simulink model "controller_dev_sg_HIL_noTP"  (R2018b)
settings: configuration reference "Physics" (kept outside this file)
model workspace (MAT data in the model file):
  m = 1000
values from neighbouring files (symbols this model uses):
  bool_activate_Vehicles : value not decoded    [controller_dev_sg.sldd]
  ModObj_ObjList_SendPort = 11004.0    [UDPPortConfig.sldd]
  ModSens_GpsSenDat_SendPort = 3002.0    [UDPPortConfig.sldd]
  sensors_freq_camera = 37.0    [controller_dev_sg.sldd]
  sensors_freq_gps = 20.0    [controller_dev_sg.sldd]
  sensors_freq_imu = 100.0    [controller_dev_sg.sldd]
  sensors_freq_lidar = 12.0    [controller_dev_sg.sldd]
  sensors_freq_radar = 20.0    [controller_dev_sg.sldd]
undefined symbols (not defined in the file or in its folder): activate_VariableFriction, C, tpa_map_Reference, tSPhysics, x0_vehiclepos_start_veh1, x0_vehiclepos_start_veh10, x0_vehiclepos_start_veh2, x0_vehiclepos_start_veh3, x0_vehiclepos_start_veh4, x0_vehiclepos_start_veh5, x0_vehiclepos_start_veh6, x0_vehiclepos_start_veh7, x0_vehiclepos_start_veh8, x0_vehiclepos_start_veh9
libraries: xpcutilitieslib x273, xpcrtudplib x215, aerolibconvert2 x48, simulink x30, etargetslib x26, speedgoatlib_IO612 x7, canmsglib x6, slrtlib x4
(part 1 of 16)
settings Model: DataDictionary=controller_dev_sg.sldd  sg_rtwmakecfg_data=_sglibc__IO61X_Library_  PauseTimes=9.280  Creator=wischnewski  LastModifiedBy=ga96wud

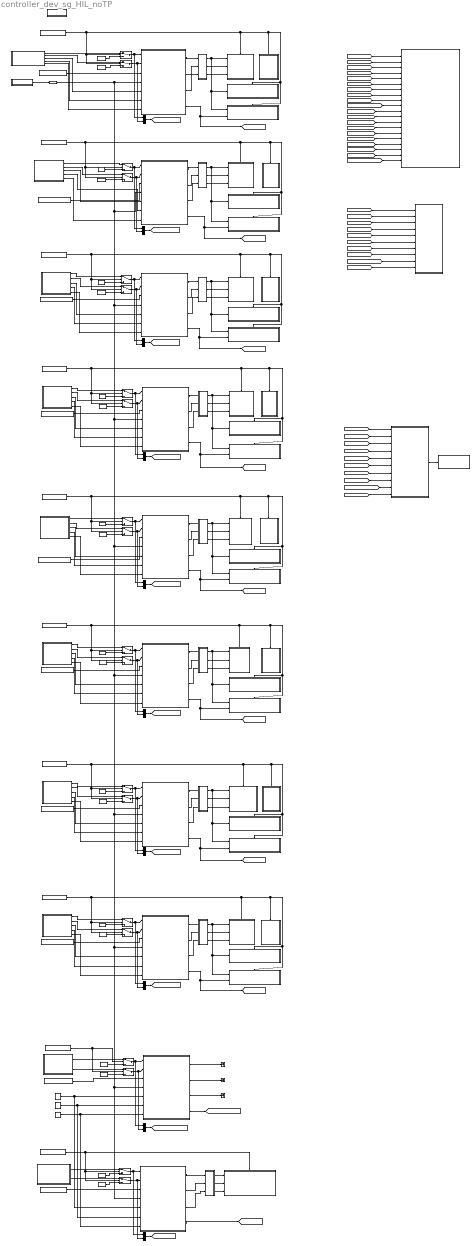
== system controller_dev_sg_HIL_noTP ==
  note: UDP to Object Detection (Object List)
  note: Roborace Vehicle on Nvidia and Speedgoat Mobile
  note: Author: Alexander Wischnewski (alexander.wischnewski@tum.de)
      | Chair of Automatic Control at TU Munich
      |
      | Description: This model uses the control software provided in vehicle dynamics control and the nonlinear single track vehicle model
      | with sensor models to simulate the example vehicle in closed loop.
  note: UDP to Unity Environment Simulation (Vehicle States)
  note: Dallara 1
  note: Configuration of Speedgoat Scopes
  note: Dallara 2
  note: Manual Steering
  note: Dallara 3
  note: Dallara 4
  note: Dallara 5
  note: Dallara 6
  note: Dallara 7
  note: Dallara 8
  Constant{,2,6,8..9,13,17,21..22,25,28,31..32} (13 alike) : Constant  Value=0
  Constant{1,3,10,12,14,18..19,23,26,29} (10 alike) : Constant  Value=-1000
  Constant11 : Constant  Value=bool_activate_Vehicles(1)  OutDataTypeStr=boolean
  Constant15 : Constant  Value=bool_activate_Vehicles(10)  OutDataTypeStr=boolean
  Constant16 : Constant  Value=bool_activate_Vehicles(3)  OutDataTypeStr=boolean
  Constant20 : Constant  Value=bool_activate_Vehicles(4)  OutDataTypeStr=boolean
  Constant24 : Constant  Value=bool_activate_Vehicles(6)  OutDataTypeStr=boolean
  Constant27 : Constant  Value=bool_activate_Vehicles(7)  OutDataTypeStr=boolean
  Constant30 : Constant  Value=bool_activate_Vehicles(8)  OutDataTypeStr=boolean
  Constant4 : Constant  Value=bool_activate_Vehicles(2)  OutDataTypeStr=boolean
  Constant5 : Constant  Value=bool_activate_Vehicles(9)  OutDataTypeStr=boolean
  Constant7 : Constant  Value=bool_activate_Vehicles(5)  OutDataTypeStr=boolean
  EnvironmentSim_Communication : Subsystem
  HardwareSetup : Subsystem
  Model{,1..8} (9 alike) : ModelReference  ModelNameDialog=convert_SimBus.slx  SimulationMode=Normal  ModelReferenceVersion=1.823
  Mux{,1..9} (10 alike) : Mux  Inputs=2
  Object List Preparation : Subsystem
  PassengerVehicle -  Manual Steering : ModelReference  ModelNameDialog=PassengerVehicle  SimulationMode=Normal  ModelReferenceVersion=1.994
  PassengerVehicle - Dallara {1..8} (8 alike) : ModelReference  ModelNameDialog=PassengerVehicle  SimulationMode=Normal  ModelReferenceVersion=1.994
  PassengerVehicle - Roborace : ModelReference  ModelNameDialog=PassengerVehicle  SimulationMode=Normal  ModelReferenceVersion=1.994
  Raptor State Machine 1 : Subsystem
  Raptor State Machine 2 : Subsystem
  Raptor State Machine 3 : Subsystem
  Raptor State Machine 4 : Subsystem
  Raptor State Machine 5 : Subsystem
  Raptor State Machine 6 : Subsystem
  Raptor State Machine 7 : Subsystem
  Raptor State Machine 8 : Subsystem
  Rate Transition5 : RateTransition
  Rx_VehicleControlCAN : Subsystem
  SpeedgoatScopes : Subsystem
  Subsystem1 : Subsystem
  Subsystem4 : Subsystem
  Switch{1..20} (20 alike) : Switch  Criteria=u2 > Threshold  Threshold=0.5
  Terminator3 : Terminator
  Terminator4 : Terminator
  Terminator5 : Terminator
  Tx_VehicleDataCAN : Subsystem
  "UDP from Control (Request for Steering Angle, Long. Force)" : Subsystem
  "UDP from Control (Request for Steering Angle, Long. Force)1" : Subsystem
  "UDP from Control (Request for Steering Angle, Long. Force)2" : Subsystem
  "UDP from Control (Request for Steering Angle, Long. Force)3" : Subsystem
  "UDP from Control (Request for Steering Angle, Long. Force)4" : Subsystem
  "UDP from Control (Request for Steering Angle, Long. Force)5" : Subsystem
  "UDP from Control (Request for Steering Angle, Long. Force)6" : Subsystem
  "UDP from Control (Request for Steering Angle, Long. Force)7" : Subsystem
  "UDP to Control (Position, IMU, Wheelspeed)" : Subsystem
  "UDP to Control (Position, IMU, Wheelspeed)1" : Subsystem
  "UDP to Control (Position, IMU, Wheelspeed)2" : Subsystem
  "UDP to Control (Position, IMU, Wheelspeed)3" : Subsystem
  "UDP to Control (Position, IMU, Wheelspeed)4" : Subsystem
  "UDP to Control (Position, IMU, Wheelspeed)5" : Subsystem
  "UDP to Control (Position, IMU, Wheelspeed)6" : Subsystem
  "UDP to Control (Position, IMU, Wheelspeed)7" : Subsystem
  "UDP to Mapping and Localization (Position, IMU, Wheelspeed)" : Subsystem
  "UDP to Mapping and Localization (Position, IMU, Wheelspeed)1" : Subsystem
  "UDP to Mapping and Localization (Position, IMU, Wheelspeed)2" : Subsystem
  "UDP to Mapping and Localization (Position, IMU, Wheelspeed)3" : Subsystem
  "UDP to Mapping and Localization (Position, IMU, Wheelspeed)4" : Subsystem
  "UDP to Mapping and Localization (Position, IMU, Wheelspeed)5" : Subsystem
  "UDP to Mapping and Localization (Position, IMU, Wheelspeed)6" : Subsystem
  "UDP to Mapping and Localization (Position, IMU, Wheelspeed)7" : Subsystem
  UDP to Object Detection : Subsystem
  "UDP to Sensors (GNSS, IMU)" : Subsystem
  "UDP to Sensors (GNSS, IMU)1" : Subsystem
  "UDP to Sensors (GNSS, IMU)2" : Subsystem
  "UDP to Sensors (GNSS, IMU)3" : Subsystem
  "UDP to Sensors (GNSS, IMU)4" : Subsystem
  "UDP to Sensors (GNSS, IMU)5" : Subsystem
  "UDP to Sensors (GNSS, IMU)6" : Subsystem
  "UDP to Sensors (GNSS, IMU)7" : Subsystem
  x0_Dallara1 : Constant  Value=[x0_vehiclepos_start_veh1 1]  VectorParams1D=off
  x0_Dallara2 : Constant  Value=[x0_vehiclepos_start_veh2 1]
  x0_Dallara3 : Constant  Value=[x0_vehiclepos_start_veh3 1]
  x0_Dallara4 : Constant  Value=[x0_vehiclepos_start_veh4 1]
  x0_Dallara5 : Constant  Value=[x0_vehiclepos_start_veh5 1]
  x0_Dallara6 : Constant  Value=[x0_vehiclepos_start_veh6 1]
  x0_Dallara7 : Constant  Value=[x0_vehiclepos_start_veh7 1]
  x0_Dallara8 : Constant  Value=[x0_vehiclepos_start_veh8 1]
  x0_DevBot : Constant  Value=[x0_vehiclepos_start_veh10 1]
  x0_ManSteer : Constant  Value=[x0_vehiclepos_start_veh9 1]
  wires:
  PassengerVehicle - Roborace/1 -> Model/1
  PassengerVehicle - Roborace/2 -> Model/2
  PassengerVehicle - Roborace/3 -> Model/3
  PassengerVehicle - Roborace/4 -> [SimRealState_RR]
  Switch3/1 -> Mux/1, PassengerVehicle - Roborace/1
  Switch5/1 -> Mux/2, PassengerVehicle - Roborace/2
  Rx_VehicleControlCAN/2(TractionForceSummedAtWheels_N) -> Switch5/1
  Constant15/1 -> Switch5/2, Switch3/2, Tx_VehicleDataCAN/Enable
  Model1/1 -> "UDP to Sensors (GNSS, IMU)"/1(VehicleSensorData), "UDP to Mapping and Localization (Position, IMU, Wheelspeed)"/1(VehicleSensorData), "UDP to Control (Position, IMU, Wheelspeed)"/1(VehicleSensorData)
  x0_Dallara2/1 -> PassengerVehicle - Dallara 2/3
  x0_ManSteer/1 -> PassengerVehicle -  Manual Steering/3
  x0_Dallara1/1 -> PassengerVehicle - Dallara 1/3
  Constant17/1 -> Switch3/3
  x0_DevBot/1 -> PassengerVehicle - Roborace/3
  Constant18/1 -> Switch5/3
  PassengerVehicle - Dallara 1/4 -> "UDP to Sensors (GNSS, IMU)"/2(SimRealState), [SimRealState_Dallara1]
  PassengerVehicle - Dallara 2/4 -> "UDP to Sensors (GNSS, IMU)1"/2(SimRealState), [SimRealState_Dallara2]
  PassengerVehicle -  Manual Steering/4 -> [SimRealState_ManualSteering]
  [SimRealState_RR] -> Object List Preparation/10(SimRealState_RR)
  [SimRealState_Dallara1] -> Object List Preparation/1(SimRealState_Dallara1)
  [SimRealState_Dallara2] -> Object List Preparation/2(SimRealState_Dallara2)
  [SimRealState_Dallara3] -> Object List Preparation/3(SimRealState_Dallara3)
  Model2/3 -> "UDP to Control (Position, IMU, Wheelspeed)1"/3(ActuatorLimitations)
  Model2/1 -> "UDP to Sensors (GNSS, IMU)1"/1(VehicleSensorData), "UDP to Mapping and Localization (Position, IMU, Wheelspeed)1"/1(VehicleSensorData), "UDP to Control (Position, IMU, Wheelspeed)1"/1(VehicleSensorData)
  Model2/2 -> "UDP to Control (Position, IMU, Wheelspeed)1"/2(VehicleSystemStatus)
  PassengerVehicle -  Manual Steering/3 -> Terminator3/1
  PassengerVehicle -  Manual Steering/2 -> Terminator5/1
  PassengerVehicle -  Manual Steering/1 -> Terminator4/1
  Object List Preparation/1(Objects) -> UDP to Object Detection/1(Objects)
  [SimRealState_RR] -> EnvironmentSim_Communication/10(SimRealState_RR)
  [SimRealState_Dallara1] -> EnvironmentSim_Communication/1(SimRealState_Dallara1)
  [SimRealState_Dallara2] -> EnvironmentSim_Communication/2(SimRealState_Dallara2)
  [SimRealState_Dallara3] -> EnvironmentSim_Communication/3(SimRealState_Dallara3)
  Constant3/1 -> Switch4/3
  Constant2/1 -> Switch2/3
  "UDP from Control (Request for Steering Angle, Long. Force)1"/1(SteeringAngleAtWheel_rad) -> Switch2/1
  "UDP from Control (Request for Steering Angle, Long. Force)1"/2(TractionForceSummedAtWheels_N) -> Switch4/1
  [SimRealState_RR] -> SpeedgoatScopes/1(SimRealState_RoboraceDB)
  [SimRealState_Dallara3] -> SpeedgoatScopes/4(SimRealState_Dallara3)
  [SimRealState_Dallara2] -> SpeedgoatScopes/3(SimRealState_Dallara2)
  [SimRealState_Dallara1] -> SpeedgoatScopes/2(SimRealState_Dallara1)
  Mux/1 -> [ControlCommand_RR]
  Mux1/1 -> [ControlCommand_Dallara1]
  Switch7/1 -> Mux1/1, PassengerVehicle - Dallara 1/1
  Switch1/1 -> Mux1/2, PassengerVehicle - Dallara 1/2
  Mux2/1 -> [ControlCommand_Dallara2]
  Switch4/1 -> Mux2/2, PassengerVehicle - Dallara 2/2
  Switch2/1 -> Mux2/1, PassengerVehicle - Dallara 2/1
  Mux3/1 -> [ControlCommand_ManualSteering]
  [ControlCommand_RR] -> SpeedgoatScopes/11(ControlCommand_RoboraceDB)
  [ControlCommand_Dallara1] -> SpeedgoatScopes/12(ControlCommand_Dallara1)
  [ControlCommand_Dallara2] -> SpeedgoatScopes/13(ControlCommand_Dallara2)
  [ControlCommand_Dallara3] -> SpeedgoatScopes/14(ControlCommand_Dallara3)
  Subsystem1/1(in_tpamapReference) -> Rate Transition5/1
  Rate Transition5/1 -> PassengerVehicle - Dallara 2/4, PassengerVehicle - Dallara 3/4, PassengerVehicle - Dallara 4/4, PassengerVehicle - Dallara 5/4, PassengerVehicle - Dallara 6/4, PassengerVehicle - Dallara 7/4, PassengerVehicle - Roborace/4, PassengerVehicle -  Manual Steering/4, PassengerVehicle - Dallara 8/4, PassengerVehicle - Dallara 1/4
  Constant11/1 -> Switch1/2, Switch7/2, "UDP to Sensors (GNSS, IMU)"/Enable, "UDP to Mapping and Localization (Position, IMU, Wheelspeed)"/Enable, Raptor State Machine 1/Enable, "UDP to Control (Position, IMU, Wheelspeed)"/Enable
  Model/1 -> Tx_VehicleDataCAN/1(VehicleSensorData)
  Model/3 -> Tx_VehicleDataCAN/3(ActuatorLimitations)
  Model/2 -> Tx_VehicleDataCAN/2(VehicleSystemStatus)
  PassengerVehicle - Dallara 1/2 -> Model1/2
  PassengerVehicle - Dallara 1/3 -> Model1/3
  Model1/3 -> "UDP to Control (Position, IMU, Wheelspeed)"/3(ActuatorLimitations)
  Model1/2 -> "UDP to Control (Position, IMU, Wheelspeed)"/2(VehicleSystemStatus)
  PassengerVehicle - Dallara 1/1 -> Model1/1
  PassengerVehicle - Dallara 2/3 -> Model2/3
  PassengerVehicle - Dallara 2/2 -> Model2/2
  PassengerVehicle - Dallara 2/1 -> Model2/1
  Rx_VehicleControlCAN/1(SteeringAngleAtWheel_rad) -> Switch3/1
  Switch12/1 -> Mux3/1, PassengerVehicle -  Manual Steering/1
  Switch13/1 -> Mux3/2, PassengerVehicle -  Manual Steering/2
  Constant6/1 -> Switch7/3
  Constant14/1 -> Switch1/3
  "UDP from Control (Request for Steering Angle, Long. Force)"/1(SteeringAngleAtWheel_rad) -> Switch7/1
  "UDP from Control (Request for Steering Angle, Long. Force)"/2(TractionForceSummedAtWheels_N) -> Switch1/1
  Constant/1 -> PassengerVehicle -  Manual Steering/5, PassengerVehicle - Roborace/5
  Constant8/1 -> PassengerVehicle -  Manual Steering/6, PassengerVehicle - Roborace/6
  Mux4/1 -> [ControlCommand_Dallara3]
  Model3/3 -> "UDP to Control (Position, IMU, Wheelspeed)2"/3(ActuatorLimitations)
  Model3/2 -> "UDP to Control (Position, IMU, Wheelspeed)2"/2(VehicleSystemStatus)
  PassengerVehicle - Dallara 3/1 -> Model3/1
  Constant16/1 -> Raptor State Machine 3/Enable, "UDP to Sensors (GNSS, IMU)2"/Enable, "UDP to Mapping and Localization (Position, IMU, Wheelspeed)2"/Enable, "UDP to Control (Position, IMU, Wheelspeed)2"/Enable, Switch9/2, Switch8/2
  PassengerVehicle - Dallara 3/2 -> Model3/2
  Switch8/1 -> Mux4/1, PassengerVehicle - Dallara 3/1
  PassengerVehicle - Dallara 3/3 -> Model3/3
  Switch9/1 -> Mux4/2, PassengerVehicle - Dallara 3/2
  Constant9/1 -> Switch8/3
  "UDP from Control (Request for Steering Angle, Long. Force)2"/2(TractionForceSummedAtWheels_N) -> Switch9/1
  Constant12/1 -> Switch9/3
  PassengerVehicle - Dallara 3/4 -> "UDP to Sensors (GNSS, IMU)2"/2(SimRealState), [SimRealState_Dallara3]
  x0_Dallara3/1 -> PassengerVehicle - Dallara 3/3
  Constant21/1 -> Switch10/3
  x0_Dallara4/1 -> PassengerVehicle - Dallara 4/3
  Switch11/1 -> Mux5/2, PassengerVehicle - Dallara 4/2
  PassengerVehicle - Dallara 4/4 -> "UDP to Sensors (GNSS, IMU)3"/2(SimRealState), [SimRealState_Dallara4]
  "UDP from Control (Request for Steering Angle, Long. Force)4"/2(TractionForceSummedAtWheels_N) -> Switch11/1
  Switch10/1 -> Mux5/1, PassengerVehicle - Dallara 4/1
  Model4/1 -> "UDP to Sensors (GNSS, IMU)3"/1(VehicleSensorData), "UDP to Mapping and Localization (Position, IMU, Wheelspeed)3"/1(VehicleSensorData), "UDP to Control (Position, IMU, Wheelspeed)3"/1(VehicleSensorData)
  PassengerVehicle - Dallara 4/2 -> Model4/2
  PassengerVehicle - Dallara 4/3 -> Model4/3
  Mux5/1 -> [ControlCommand_Dallara4]
  "UDP from Control (Request for Steering Angle, Long. Force)4"/1(SteeringAngleAtWheel_rad) -> Switch10/1
  Model4/2 -> "UDP to Control (Position, IMU, Wheelspeed)3"/2(VehicleSystemStatus)
  Model4/3 -> "UDP to Control (Position, IMU, Wheelspeed)3"/3(ActuatorLimitations)
  Constant19/1 -> Switch11/3
  PassengerVehicle - Dallara 4/1 -> Model4/1
  [SimRealState_Dallara4] -> SpeedgoatScopes/5(SimRealState_Dallara4)
  [ControlCommand_Dallara4] -> SpeedgoatScopes/15(ControlCommand_Dallara4)
  [SimRealState_Dallara4] -> EnvironmentSim_Communication/4(SimRealState_Dallara4)
  [SimRealState_Dallara4] -> Object List Preparation/4(SimRealState_Dallara4)
  Constant10/1 -> Switch13/3
  Constant5/1 -> Switch12/2, Switch13/2
  Subsystem4/1(SteeringWheelAngle_rad) -> Switch12/1
  Constant13/1 -> Switch12/3
  Subsystem4/2(TractionForceSummedAtWheels_N) -> Switch13/1
  "UDP from Control (Request for Steering Angle, Long. Force)"/3(ThrottleRequest_perc) -> PassengerVehicle - Dallara 1/5
  "UDP from Control (Request for Steering Angle, Long. Force)"/4(GearRequest) -> PassengerVehicle - Dallara 1/6
  "UDP from Control (Request for Steering Angle, Long. Force)"/5(BrakeRequest_bar) -> PassengerVehicle - Dallara 1/7
  "UDP from Control (Request for Steering Angle, Long. Force)1"/3(ThrottleRequest_perc) -> PassengerVehicle - Dallara 2/5
  "UDP from Control (Request for Steering Angle, Long. Force)1"/4(GearRequest) -> PassengerVehicle - Dallara 2/6
  "UDP from Control (Request for Steering Angle, Long. Force)1"/5(BrakeRequest_bar) -> PassengerVehicle - Dallara 2/7
  "UDP from Control (Request for Steering Angle, Long. Force)2"/1(SteeringAngleAtWheel_rad) -> Switch8/1
  "UDP from Control (Request for Steering Angle, Long. Force)2"/3(ThrottleRequest_perc) -> PassengerVehicle - Dallara 3/5
  "UDP from Control (Request for Steering Angle, Long. Force)2"/4(GearRequest) -> PassengerVehicle - Dallara 3/6
  "UDP from Control (Request for Steering Angle, Long. Force)2"/5(BrakeRequest_bar) -> PassengerVehicle - Dallara 3/7
  "UDP from Control (Request for Steering Angle, Long. Force)4"/3(ThrottleRequest_perc) -> PassengerVehicle - Dallara 4/5
  "UDP from Control (Request for Steering Angle, Long. Force)4"/4(GearRequest) -> PassengerVehicle - Dallara 4/6
  "UDP from Control (Request for Steering Angle, Long. Force)4"/5(BrakeRequest_bar) -> PassengerVehicle - Dallara 4/7
  PassengerVehicle - Dallara 5/4 -> "UDP to Sensors (GNSS, IMU)4"/2(SimRealState), [SimRealState_Dallara5]
  PassengerVehicle - Dallara 5/2 -> Model5/2
  "UDP from Control (Request for Steering Angle, Long. Force)3"/3(ThrottleRequest_perc) -> PassengerVehicle - Dallara 5/5
  Constant22/1 -> Switch6/3
  "UDP from Control (Request for Steering Angle, Long. Force)3"/5(BrakeRequest_bar) -> PassengerVehicle - Dallara 5/7
  Model5/2 -> "UDP to Control (Position, IMU, Wheelspeed)4"/2(VehicleSystemStatus)
  Constant7/1 -> Raptor State Machine 5/Enable, "UDP to Sensors (GNSS, IMU)4"/Enable, "UDP to Mapping and Localization (Position, IMU, Wheelspeed)4"/Enable, "UDP to Control (Position, IMU, Wheelspeed)4"/Enable, Switch14/2, Switch6/2
  Model5/3 -> "UDP to Control (Position, IMU, Wheelspeed)4"/3(ActuatorLimitations)
  PassengerVehicle - Dallara 5/3 -> Model5/3
  Mux6/1 -> [ControlCommand_Dallara5]
  Switch6/1 -> Mux6/1, PassengerVehicle - Dallara 5/1
  Model5/1 -> "UDP to Control (Position, IMU, Wheelspeed)4"/1(VehicleSensorData), "UDP to Sensors (GNSS, IMU)4"/1(VehicleSensorData), "UDP to Mapping and Localization (Position, IMU, Wheelspeed)4"/1(VehicleSensorData)
  Constant1/1 -> Switch14/3
  "UDP from Control (Request for Steering Angle, Long. Force)3"/1(SteeringAngleAtWheel_rad) -> Switch6/1
  "UDP from Control (Request for Steering Angle, Long. Force)3"/4(GearRequest) -> PassengerVehicle - Dallara 5/6
  PassengerVehicle - Dallara 5/1 -> Model5/1
  Switch14/1 -> Mux6/2, PassengerVehicle - Dallara 5/2
  x0_Dallara5/1 -> PassengerVehicle - Dallara 5/3
  "UDP from Control (Request for Steering Angle, Long. Force)3"/2(TractionForceSummedAtWheels_N) -> Switch14/1
  PassengerVehicle - Dallara 6/4 -> "UDP to Sensors (GNSS, IMU)5"/2(SimRealState), [SimRealState_Dallara6]
  PassengerVehicle - Dallara 6/2 -> Model6/2
  "UDP from Control (Request for Steering Angle, Long. Force)5"/3(ThrottleRequest_perc) -> PassengerVehicle - Dallara 6/5
  Constant25/1 -> Switch15/3
  "UDP from Control (Request for Steering Angle, Long. Force)5"/5(BrakeRequest_bar) -> PassengerVehicle - Dallara 6/7
  Model6/2 -> "UDP to Control (Position, IMU, Wheelspeed)5"/2(VehicleSystemStatus)
  Constant24/1 -> Raptor State Machine 6/Enable, "UDP to Sensors (GNSS, IMU)5"/Enable, "UDP to Mapping and Localization (Position, IMU, Wheelspeed)5"/Enable, "UDP to Control (Position, IMU, Wheelspeed)5"/Enable, Switch16/2, Switch15/2
  Model6/3 -> "UDP to Control (Position, IMU, Wheelspeed)5"/3(ActuatorLimitations)
  PassengerVehicle - Dallara 6/3 -> Model6/3
  Mux7/1 -> [ControlCommand_Dallara6]
  Switch15/1 -> Mux7/1, PassengerVehicle - Dallara 6/1
  Model6/1 -> "UDP to Control (Position, IMU, Wheelspeed)5"/1(VehicleSensorData), "UDP to Sensors (GNSS, IMU)5"/1(VehicleSensorData), "UDP to Mapping and Localization (Position, IMU, Wheelspeed)5"/1(VehicleSensorData)
  Constant23/1 -> Switch16/3
  "UDP from Control (Request for Steering Angle, Long. Force)5"/1(SteeringAngleAtWheel_rad) -> Switch15/1
  "UDP from Control (Request for Steering Angle, Long. Force)5"/4(GearRequest) -> PassengerVehicle - Dallara 6/6
  PassengerVehicle - Dallara 6/1 -> Model6/1
  Switch16/1 -> Mux7/2, PassengerVehicle - Dallara 6/2
  x0_Dallara6/1 -> PassengerVehicle - Dallara 6/3
  "UDP from Control (Request for Steering Angle, Long. Force)5"/2(TractionForceSummedAtWheels_N) -> Switch16/1
  PassengerVehicle - Dallara 7/4 -> "UDP to Sensors (GNSS, IMU)6"/2(SimRealState), [SimRealState_Dallara7]
  PassengerVehicle - Dallara 7/2 -> Model7/2
  "UDP from Control (Request for Steering Angle, Long. Force)6"/3(ThrottleRequest_perc) -> PassengerVehicle - Dallara 7/5
  Constant28/1 -> Switch17/3
  "UDP from Control (Request for Steering Angle, Long. Force)6"/5(BrakeRequest_bar) -> PassengerVehicle - Dallara 7/7
  Model7/2 -> "UDP to Control (Position, IMU, Wheelspeed)6"/2(VehicleSystemStatus)
  Constant27/1 -> Raptor State Machine 7/Enable, "UDP to Sensors (GNSS, IMU)6"/Enable, "UDP to Mapping and Localization (Position, IMU, Wheelspeed)6"/Enable, "UDP to Control (Position, IMU, Wheelspeed)6"/Enable, Switch18/2, Switch17/2
  Model7/3 -> "UDP to Control (Position, IMU, Wheelspeed)6"/3(ActuatorLimitations)
  PassengerVehicle - Dallara 7/3 -> Model7/3
  Mux8/1 -> [ControlCommand_Dallara7]
  Switch17/1 -> Mux8/1, PassengerVehicle - Dallara 7/1
  Model7/1 -> "UDP to Sensors (GNSS, IMU)6"/1(VehicleSensorData), "UDP to Mapping and Localization (Position, IMU, Wheelspeed)6"/1(VehicleSensorData), "UDP to Control (Position, IMU, Wheelspeed)6"/1(VehicleSensorData)
  Constant26/1 -> Switch18/3
  "UDP from Control (Request for Steering Angle, Long. Force)6"/1(SteeringAngleAtWheel_rad) -> Switch17/1
  "UDP from Control (Request for Steering Angle, Long. Force)6"/4(GearRequest) -> PassengerVehicle - Dallara 7/6
  PassengerVehicle - Dallara 7/1 -> Model7/1
  Switch18/1 -> Mux8/2, PassengerVehicle - Dallara 7/2
  x0_Dallara7/1 -> PassengerVehicle - Dallara 7/3
  "UDP from Control (Request for Steering Angle, Long. Force)6"/2(TractionForceSummedAtWheels_N) -> Switch18/1
  PassengerVehicle - Dallara 8/4 -> "UDP to Sensors (GNSS, IMU)7"/2(SimRealState), [SimRealState_Dallara8]
  PassengerVehicle - Dallara 8/2 -> Model8/2
  "UDP from Control (Request for Steering Angle, Long. Force)7"/3(ThrottleRequest_perc) -> PassengerVehicle - Dallara 8/5
  Constant31/1 -> Switch19/3
  "UDP from Control (Request for Steering Angle, Long. Force)7"/5(BrakeRequest_bar) -> PassengerVehicle - Dallara 8/7
  Model8/2 -> "UDP to Control (Position, IMU, Wheelspeed)7"/2(VehicleSystemStatus)
  Constant30/1 -> Raptor State Machine 8/Enable, "UDP to Sensors (GNSS, IMU)7"/Enable, "UDP to Mapping and Localization (Position, IMU, Wheelspeed)7"/Enable, "UDP to Control (Position, IMU, Wheelspeed)7"/Enable, Switch20/2, Switch19/2
  Model8/3 -> "UDP to Control (Position, IMU, Wheelspeed)7"/3(ActuatorLimitations)
  PassengerVehicle - Dallara 8/3 -> Model8/3
  Mux9/1 -> [ControlCommand_Dallara8]
  Switch19/1 -> Mux9/1, PassengerVehicle - Dallara 8/1
  Model8/1 -> "UDP to Control (Position, IMU, Wheelspeed)7"/1(VehicleSensorData), "UDP to Sensors (GNSS, IMU)7"/1(VehicleSensorData), "UDP to Mapping and Localization (Position, IMU, Wheelspeed)7"/1(VehicleSensorData)
  Constant29/1 -> Switch20/3
  "UDP from Control (Request for Steering Angle, Long. Force)7"/1(SteeringAngleAtWheel_rad) -> Switch19/1
  "UDP from Control (Request for Steering Angle, Long. Force)7"/4(GearRequest) -> PassengerVehicle - Dallara 8/6
  PassengerVehicle - Dallara 8/1 -> Model8/1
  Switch20/1 -> Mux9/2, PassengerVehicle - Dallara 8/2
  x0_Dallara8/1 -> PassengerVehicle - Dallara 8/3
  "UDP from Control (Request for Steering Angle, Long. Force)7"/2(TractionForceSummedAtWheels_N) -> Switch20/1
  [ControlCommand_ManualSteering] -> SpeedgoatScopes/20(ControlCommand_ManSteer)
  [ControlCommand_Dallara8] -> SpeedgoatScopes/19(ControlCommand_Dallara8)
  [ControlCommand_Dallara7] -> SpeedgoatScopes/18(ControlCommand_Dallara7)
  [ControlCommand_Dallara6] -> SpeedgoatScopes/17(ControlCommand_Dallara6)
  [ControlCommand_Dallara5] -> SpeedgoatScopes/16(ControlCommand_Dallara5)
  [SimRealState_ManualSteering] -> SpeedgoatScopes/10(SimRealState_ManSteer)
  [SimRealState_Dallara8] -> SpeedgoatScopes/9(SimRealState_Dallara8)
  [SimRealState_Dallara7] -> SpeedgoatScopes/8(SimRealState_Dallara7)
  [SimRealState_Dallara6] -> SpeedgoatScopes/7(SimRealState_Dallara6)
  [SimRealState_Dallara5] -> SpeedgoatScopes/6(SimRealState_Dallara5)
  [SimRealState_ManualSteering] -> EnvironmentSim_Communication/9(SimRealState_ManSteer)
  [SimRealState_Dallara8] -> EnvironmentSim_Communication/8(SimRealState_Dallara8)
  [SimRealState_Dallara5] -> EnvironmentSim_Communication/5(SimRealState_Dallara5)
  [SimRealState_Dallara6] -> EnvironmentSim_Communication/6(SimRealState_Dallara6)
  [SimRealState_Dallara7] -> EnvironmentSim_Communication/7(SimRealState_Dallara7)
  [SimRealState_Dallara5] -> Object List Preparation/5(SimRealState_Dallara5)
  [SimRealState_Dallara6] -> Object List Preparation/6(SimRealState_Dallara6)
  [SimRealState_Dallara7] -> Object List Preparation/7(SimRealState_Dallara7)
  [SimRealState_Dallara8] -> Object List Preparation/8(SimRealState_Dallara8)
  [SimRealState_ManualSteering] -> Object List Preparation/9(SimRealState_ManSteer)
  Constant20/1 -> "UDP to Sensors (GNSS, IMU)3"/Enable, "UDP to Mapping and Localization (Position, IMU, Wheelspeed)3"/Enable, Raptor State Machine 4/Enable, "UDP to Control (Position, IMU, Wheelspeed)3"/Enable, Switch11/2, Switch10/2
  Constant32/1 -> PassengerVehicle -  Manual Steering/7, PassengerVehicle - Roborace/7
  Model3/1 -> "UDP to Control (Position, IMU, Wheelspeed)2"/1(VehicleSensorData), "UDP to Sensors (GNSS, IMU)2"/1(VehicleSensorData), "UDP to Mapping and Localization (Position, IMU, Wheelspeed)2"/1(VehicleSensorData)
  Constant4/1 -> Raptor State Machine 2/Enable, "UDP to Sensors (GNSS, IMU)1"/Enable, "UDP to Mapping and Localization (Position, IMU, Wheelspeed)1"/Enable, "UDP to Control (Position, IMU, Wheelspeed)1"/Enable, Switch4/2, Switch2/2

== system controller_dev_sg_HIL_noTP/EnvironmentSim_Communication ==
  SimRealState_Dallara1 : Inport
  SimRealState_Dallara2 : Inport  Port=2
  SimRealState_Dallara3 : Inport  Port=3
  SimRealState_Dallara4 : Inport  Port=4
  SimRealState_Dallara5 : Inport  Port=5
  SimRealState_Dallara6 : Inport  Port=6
  SimRealState_Dallara7 : Inport  Port=7
  SimRealState_Dallara8 : Inport  Port=8
  SimRealState_ManSteer : Inport  Port=9
  SimRealState_RR : Inport  Port=10
  Constant : Constant  Value=zeros(34,1)
  Constant1 : Constant  Value=bool_activate_Vehicles(2)  OutDataTypeStr=boolean
  Constant15 : Constant  Value=bool_activate_Vehicles(1)  OutDataTypeStr=boolean
  Constant2 : Constant  Value=bool_activate_Vehicles(3)  OutDataTypeStr=boolean
  Constant3 : Constant  Value=bool_activate_Vehicles(4)  OutDataTypeStr=boolean
  Constant4 : Constant  Value=bool_activate_Vehicles(5)  OutDataTypeStr=boolean
  Constant5 : Constant  Value=bool_activate_Vehicles(6)  OutDataTypeStr=boolean
  Constant6 : Constant  Value=bool_activate_Vehicles(7)  OutDataTypeStr=boolean
  Constant7 : Constant  Value=bool_activate_Vehicles(8)  OutDataTypeStr=boolean
  Constant8 : Constant  Value=bool_activate_Vehicles(9)  OutDataTypeStr=boolean
  Constant9 : Constant  Value=bool_activate_Vehicles(10)  OutDataTypeStr=boolean
  Matrix Concatenate : Concatenate  NumInputs=10  Mode=Multidimensional array
  Subsystem : Subsystem  TreatAsAtomicUnit=on  SystemSampleTime=0.02
  Switch{,1..9} (10 alike) : Switch  Criteria=u2 > Threshold  Threshold=0.5
  prepare data for sending : Subsystem
  prepare data for sending1 : Subsystem
  prepare data for sending2 : Subsystem
  prepare data for sending3 : Subsystem
  prepare data for sending4 : Subsystem
  prepare data for sending5 : Subsystem
  prepare data for sending6 : Subsystem
  prepare data for sending7 : Subsystem
  prepare data for sending8 : Subsystem
  prepare data for sending9 : Subsystem
  wires:
  prepare data for sending/1(Out1) -> Switch/1
  Constant15/1 -> Switch/2
  Constant1/1 -> Switch1/2
  Constant2/1 -> Switch2/2
  Constant3/1 -> Switch3/2
  prepare data for sending2/1(Out1) -> Switch2/1
  prepare data for sending1/1(Out1) -> Switch1/1
  prepare data for sending3/1(Out1) -> Switch3/1
  Switch/1 -> Matrix Concatenate/1
  Switch1/1 -> Matrix Concatenate/2
  Switch2/1 -> Matrix Concatenate/3
  Switch3/1 -> Matrix Concatenate/4
  Matrix Concatenate/1 -> Subsystem/1(data)
  prepare data for sending4/1(Out1) -> Switch4/1
  Switch4/1 -> Matrix Concatenate/5
  Switch5/1 -> Matrix Concatenate/6
  prepare data for sending5/1(Out1) -> Switch5/1
  Constant5/1 -> Switch5/2
  Constant4/1 -> Switch4/2
  prepare data for sending9/1(Out1) -> Switch9/1
  Constant8/1 -> Switch8/2
  Constant/1 -> Switch1/3, Switch2/3, Switch4/3, Switch8/3, Switch9/3, Switch7/3, Switch6/3, Switch5/3, Switch3/3, Switch/3
  prepare data for sending8/1(Out1) -> Switch8/1
  Constant7/1 -> Switch7/2
  prepare data for sending6/1(Out1) -> Switch6/1
  Constant9/1 -> Switch9/2
  Constant6/1 -> Switch6/2
  prepare data for sending7/1(Out1) -> Switch7/1
  Switch6/1 -> Matrix Concatenate/7
  Switch7/1 -> Matrix Concatenate/8
  Switch8/1 -> Matrix Concatenate/9
  Switch9/1 -> Matrix Concatenate/10
  SimRealState_Dallara1/1 -> prepare data for sending/1(In1)
  SimRealState_Dallara2/1 -> prepare data for sending1/1(In1)
  SimRealState_Dallara3/1 -> prepare data for sending2/1(In1)
  SimRealState_Dallara4/1 -> prepare data for sending3/1(In1)
  SimRealState_Dallara5/1 -> prepare data for sending4/1(In1)
  SimRealState_Dallara6/1 -> prepare data for sending5/1(In1)
  SimRealState_Dallara7/1 -> prepare data for sending6/1(In1)
  SimRealState_Dallara8/1 -> prepare data for sending7/1(In1)
  SimRealState_ManSteer/1 -> prepare data for sending8/1(In1)
  SimRealState_RR/1 -> prepare data for sending9/1(In1)

== system controller_dev_sg_HIL_noTP/HardwareSetup ==
  CAN Setup : speedgoatlib_IO612/CAN Setup  id=1  drvLtr=C:  PCISlot=[5 0]  port1=CAN (HS)  port2=CAN (HS)  port3=Disable  port4=Disable  opModeCAN1=Highspeed (HS)  bdrCAN1=1 MBaud  usrBdrCAN1=[5, 1, 13, 2]  stdAccMaskCAN1=[0, 0]  extAccMaskCAN1=[0, 0]  opModeCAN2=Highspeed (HS)  bdrCAN2=1 MBaud  usrBdrCAN2=[5, 1, 13, 2]  stdAccMaskCAN2=[0, 0]  extAccMaskCAN2=[0, 0]  opModeCAN3=Highspeed (HS)  bdrCAN3=1 MBaud  usrBdrCAN3=[5, 1, 13, 2]  stdAccMaskCAN3=[0, 0]  extAccMaskCAN3=[0, 0]  opModeCAN4=Highspeed (HS)  bdrCAN4=1 MBaud  usrBdrCAN4=[5, 1, 13, 2]  stdAccMaskCAN4=[0, 0]  extAccMaskCAN4=[0, 0]  initStruct=[]  termStruct=[]  protl=IO612  qtyMod=1  chNo=[1, 2, 3, 4]  ptTypes=[1, 1, 1, 1]  protlHelpIdx=[0, 1, 2, 3]  isFDMod=0
      settings: SourceProductName=Simulink Real-Time: Speedgoat I/O Driver Library
  "Real-time UDP Configuration " : xpcrtudplib/UDP Configure  Priority=1  IpAddress=192.168.0.2  SubnetMask=255.255.255.0  Gateway=0.0.0.0  PciBus=14  PciSlot=0  PciFunction=0  ID=3  tune=0  disable=off  enableMulticast=off  MulticastIpAddress={}  MulticastMask={}
      settings: SourceProductName=Simulink Real-Time  SourceProductBaseCode=XP
  Real-time UDP Configuration 1 : xpcrtudplib/UDP Configure  Priority=1  IpAddress=10.0.0.20  SubnetMask=255.255.255.0  Gateway=0.0.0.0  PciBus=13  PciSlot=0  PciFunction=0  ID=3  tune=0  disable=off  enableMulticast=off  MulticastIpAddress={}  MulticastMask={}
      settings: SourceProductName=Simulink Real-Time  SourceProductBaseCode=XP

== system controller_dev_sg_HIL_noTP/Object List Preparation ==
  SimRealState_Dallara1 : Inport
  SimRealState_Dallara2 : Inport  Port=2
  SimRealState_Dallara3 : Inport  Port=3
  SimRealState_Dallara4 : Inport  Port=4
  SimRealState_Dallara5 : Inport  Port=5
  SimRealState_Dallara6 : Inport  Port=6
  SimRealState_Dallara7 : Inport  Port=7
  SimRealState_Dallara8 : Inport  Port=8
  SimRealState_ManSteer : Inport  Port=9
  SimRealState_RR : Inport  Port=10
  Bus Creator{,1..2,4..11} (11 alike) : BusCreator  Inputs=7
  Bus Creator3 : BusCreator  Inputs=10
  Bus Selector{,1..9} (10 alike) : BusSelector  OutputSignals=x_m,y_m,psi_rad,vx_mps,vy_mps,dPsi_radps
  Constant : Constant  Value=99
  Constant1 : Constant  Value=bool_activate_Vehicles(1)
  Constant{5..10} (6 alike) : Constant  Value=0
  Constant11 : Constant  Value=bool_activate_Vehicles(5)
  Constant12 : Constant  Value=bool_activate_Vehicles(6)
  Constant13 : Constant  Value=bool_activate_Vehicles(9)
  Constant14 : Constant  Value=bool_activate_Vehicles(10)
  Constant15 : Constant  Value=bool_activate_Vehicles(7)
  Constant16 : Constant  Value=bool_activate_Vehicles(8)
  Constant2 : Constant  Value=bool_activate_Vehicles(2)
  Constant3 : Constant  Value=bool_activate_Vehicles(3)
  Constant4 : Constant  Value=bool_activate_Vehicles(4)
  Switch{1..10} (10 alike) : Switch  Criteria=u2 > Threshold  Threshold=0.5
  const : Constant
  const1 : Constant  Value=2
  const2 : Constant  Value=3
  const3 : Constant  Value=4
  const4 : Constant  Value=5
  const5 : Constant  Value=6
  const6 : Constant  Value=7
  const7 : Constant  Value=8
  const8 : Constant  Value=9
  const9 : Constant  Value=10
  Objects : Outport
  wires:
  Constant1/1 -> Switch5/2
  Switch8/1 -> Bus Creator3/3  "Object_3"
  Switch9/1 -> Bus Creator3/4  "Object_4"
  Bus Creator4/1 -> Switch5/1  "Object_1"
  Switch5/1 -> Bus Creator3/1  "Object_1"
  Constant2/1 -> Switch7/2
  Constant3/1 -> Switch8/2
  Constant4/1 -> Switch9/2
  Bus Selector/6 -> Bus Creator4/7  "<dPsi_radps>"
  Bus Selector/5 -> Bus Creator4/6  "<vy_mps>"
  Bus Selector/4 -> Bus Creator4/5  "<vx_mps>"
  Bus Selector/3 -> Bus Creator4/4  "<psi_rad>"
  Bus Selector/2 -> Bus Creator4/3  "<y_m>"
  Bus Selector/1 -> Bus Creator4/2  "<x_m>"
  const/1 -> Bus Creator4/1  "vehicle ID"
  Constant/1 -> Bus Creator/1  "vehicle ID"
  Constant5/1 -> Bus Creator/2  "x_m"
  Constant9/1 -> Bus Creator/3  "y_m"
  Constant6/1 -> Bus Creator/4  "psi_rad"
  Constant7/1 -> Bus Creator/5  "vx_mps"
  Constant8/1 -> Bus Creator/6  "vy_mps"
  Constant10/1 -> Bus Creator/7  "dPsi_radps"
  Bus Selector3/2 -> Bus Creator1/3  "<y_m>"
  const1/1 -> Bus Creator1/1  "vehicle ID"
  Bus Selector3/3 -> Bus Creator1/4  "<psi_rad>"
  Bus Selector3/4 -> Bus Creator1/5  "<vx_mps>"
  Bus Creator1/1 -> Switch7/1  "Object_1"
  Bus Selector3/5 -> Bus Creator1/6  "<vy_mps>"
  Bus Selector3/1 -> Bus Creator1/2  "<x_m>"
  Bus Selector3/6 -> Bus Creator1/7  "<dPsi_radps>"
  Bus Selector1/6 -> Bus Creator5/7  "<dPsi_radps>"
  Bus Selector1/4 -> Bus Creator5/5  "<vx_mps>"
  Bus Selector1/5 -> Bus Creator5/6  "<vy_mps>"
  Bus Selector1/3 -> Bus Creator5/4  "<psi_rad>"
  Bus Selector1/2 -> Bus Creator5/3  "<y_m>"
  Bus Creator5/1 -> Switch8/1  "Object_1"
  const2/1 -> Bus Creator5/1  "vehicle ID"
  Bus Selector1/1 -> Bus Creator5/2  "<x_m>"
  Switch7/1 -> Bus Creator3/2  "Object_2"
  const3/1 -> Bus Creator2/1  "vehicle ID"
  Bus Selector2/1 -> Bus Creator2/2  "<x_m>"
  Bus Selector2/3 -> Bus Creator2/4  "<psi_rad>"
  Bus Selector2/5 -> Bus Creator2/6  "<vy_mps>"
  Bus Selector2/6 -> Bus Creator2/7  "<dPsi_radps>"
  Bus Selector2/2 -> Bus Creator2/3  "<y_m>"
  Bus Selector2/4 -> Bus Creator2/5  "<vx_mps>"
  Bus Creator2/1 -> Switch9/1  "Object_1"
  Bus Creator3/1 -> Objects/1
  Bus Selector4/3 -> Bus Creator6/4  "<psi_rad>"
  Bus Creator6/1 -> Switch1/1  "Object_1"
  Bus Selector4/6 -> Bus Creator6/7  "<dPsi_radps>"
  Bus Selector4/1 -> Bus Creator6/2  "<x_m>"
  Bus Selector4/4 -> Bus Creator6/5  "<vx_mps>"
  Switch1/1 -> Bus Creator3/5  "Object_5"
  const4/1 -> Bus Creator6/1  "vehicle ID"
  Bus Selector4/2 -> Bus Creator6/3  "<y_m>"
  Constant11/1 -> Switch1/2
  Bus Selector4/5 -> Bus Creator6/6  "<vy_mps>"
  Constant12/1 -> Switch2/2
  Bus Selector5/2 -> Bus Creator7/3  "<y_m>"
  Bus Selector5/5 -> Bus Creator7/6  "<vy_mps>"
  Bus Selector5/4 -> Bus Creator7/5  "<vx_mps>"
  const5/1 -> Bus Creator7/1  "vehicle ID"
  Bus Selector5/3 -> Bus Creator7/4  "<psi_rad>"
  Bus Creator7/1 -> Switch2/1  "Object_1"
  Bus Selector5/6 -> Bus Creator7/7  "<dPsi_radps>"
  Bus Selector5/1 -> Bus Creator7/2  "<x_m>"
  Switch2/1 -> Bus Creator3/6  "Object_6"
  Bus Selector6/5 -> Bus Creator9/6  "<vy_mps>"
  Bus Selector9/6 -> Bus Creator11/7  "<dPsi_radps>"
  Bus Selector9/2 -> Bus Creator11/3  "<y_m>"
  Bus Selector9/1 -> Bus Creator11/2  "<x_m>"
  Bus Selector6/2 -> Bus Creator9/3  "<y_m>"
  Bus Selector9/4 -> Bus Creator11/5  "<vx_mps>"
  const9/1 -> Bus Creator11/1  "vehicle ID"
  Bus Selector9/5 -> Bus Creator11/6  "<vy_mps>"
  Constant13/1 -> Switch3/2
  const8/1 -> Bus Creator10/1  "vehicle ID"
  Bus Selector7/1 -> Bus Creator8/2  "<x_m>"
  Bus Selector8/4 -> Bus Creator10/5  "<vx_mps>"
  const7/1 -> Bus Creator8/1  "vehicle ID"
  Bus Selector8/3 -> Bus Creator10/4  "<psi_rad>"
  Bus Selector7/4 -> Bus Creator8/5  "<vx_mps>"
  Bus Selector8/2 -> Bus Creator10/3  "<y_m>"
  Bus Selector8/5 -> Bus Creator10/6  "<vy_mps>"
  Bus Selector6/3 -> Bus Creator9/4  "<psi_rad>"
  Bus Creator8/1 -> Switch10/1  "Object_1"
  Bus Creator9/1 -> Switch6/1  "Object_1"
  Bus Selector8/1 -> Bus Creator10/2  "<x_m>"
  Bus Creator10/1 -> Switch3/1  "Object_1"
  Bus Creator11/1 -> Switch4/1  "Object_1"
  Bus Selector7/2 -> Bus Creator8/3  "<y_m>"
  Bus Selector7/3 -> Bus Creator8/4  "<psi_rad>"
  Bus Selector7/6 -> Bus Creator8/7  "<dPsi_radps>"
  Constant14/1 -> Switch4/2
  Bus Selector6/1 -> Bus Creator9/2  "<x_m>"
  Bus Selector6/6 -> Bus Creator9/7  "<dPsi_radps>"
  Bus Selector8/6 -> Bus Creator10/7  "<dPsi_radps>"
  Bus Selector9/3 -> Bus Creator11/4  "<psi_rad>"
  Bus Selector7/5 -> Bus Creator8/6  "<vy_mps>"
  const6/1 -> Bus Creator9/1  "vehicle ID"
  Constant16/1 -> Switch10/2
  Bus Selector6/4 -> Bus Creator9/5  "<vx_mps>"
  Bus Creator/1 -> Switch4/3, Switch3/3, Switch10/3, Switch6/3, Switch2/3, Switch1/3, Switch9/3, Switch8/3, Switch7/3, Switch5/3
  Constant15/1 -> Switch6/2
  Switch6/1 -> Bus Creator3/7  "Object_7"
  Switch10/1 -> Bus Creator3/8  "Object_8"
  Switch3/1 -> Bus Creator3/9  "Object_9"
  Switch4/1 -> Bus Creator3/10  "Object_10"
  SimRealState_Dallara1/1 -> Bus Selector/1
  SimRealState_Dallara2/1 -> Bus Selector3/1
  SimRealState_Dallara3/1 -> Bus Selector1/1
  SimRealState_Dallara4/1 -> Bus Selector2/1
  SimRealState_Dallara5/1 -> Bus Selector4/1
  SimRealState_Dallara6/1 -> Bus Selector5/1
  SimRealState_Dallara7/1 -> Bus Selector6/1
  SimRealState_Dallara8/1 -> Bus Selector7/1
  SimRealState_ManSteer/1 -> Bus Selector8/1
  SimRealState_RR/1 -> Bus Selector9/1

== system controller_dev_sg_HIL_noTP/Raptor State Machine 1 ==
  Enable : EnablePort
  Byte Unpack : etargetslib/Byte Unpack  dimensions={[1],[1],[1],[1]}  datatypes={'uint8','uint8','uint8','uint8'}  byteAlign=1
  Model9 : ModelReference  ModelNameDialog=RaptorStateMachine.slx  SimulationMode=Normal  ModelReferenceVersion=1.25
  Terminator : Terminator
  UDP Receive : xpcrtudplib/UDP Receive  ipAddressVal=10.0.0.20  localPort=ModCtrl_RaptorCommandVeh1_RcvPort  rcvWidth=4  rcvFmAny=on  fmAddress=10.0.0.1  rcvMulticast=off  multicastAddress={}  maxUDPQueue=8  sampleTime=-1
      settings: SourceProductName=Simulink Real-Time
  UDP Send1 : xpcrtudplib/UDP Send  ipAddressVal=10.0.0.20  localPort=40600  toAddress=10.0.0.11  toPort=ModCtrl_RaptorState_SendPort  sampleTime=-1
      settings: SourceProductName=Simulink Real-Time  SourceProductBaseCode=XP
  Width : Width
  wires:
  UDP Receive/2 -> Terminator/1
  UDP Receive/1 -> Byte Unpack/1
  Byte Unpack/3 -> Model9/3
  Byte Unpack/1 -> Model9/1
  Model9/1 -> Width/1, UDP Send1/1
  Byte Unpack/2 -> Model9/2
  Width/1 -> UDP Send1/2
  Byte Unpack/4 -> Model9/4

== system controller_dev_sg_HIL_noTP/Raptor State Machine 2 ==
  Enable : EnablePort
  Byte Unpack1 : etargetslib/Byte Unpack  dimensions={[1],[1],[1],[1]}  datatypes={'uint8','uint8','uint8','uint8'}  byteAlign=1
  Model10 : ModelReference  ModelNameDialog=RaptorStateMachine.slx  SimulationMode=Normal  ModelReferenceVersion=1.25
  Terminator1 : Terminator
  UDP Receive1 : xpcrtudplib/UDP Receive  ipAddressVal=10.0.0.20  localPort=ModCtrl_RaptorCommandVeh2_RcvPort  rcvWidth=4  rcvFmAny=on  fmAddress=10.0.0.1  rcvMulticast=off  multicastAddress={}  maxUDPQueue=8  sampleTime=-1
      settings: SourceProductName=Simulink Real-Time
  UDP Send2 : xpcrtudplib/UDP Send  ipAddressVal=10.0.0.20  localPort=40601  toAddress=10.0.0.12  toPort=ModCtrl_RaptorState_SendPort  sampleTime=-1
      settings: SourceProductName=Simulink Real-Time  SourceProductBaseCode=XP
  Width1 : Width
  wires:
  Model10/1 -> Width1/1, UDP Send2/1
  Width1/1 -> UDP Send2/2
  Byte Unpack1/1 -> Model10/1
  Byte Unpack1/2 -> Model10/2
  UDP Receive1/2 -> Terminator1/1
  Byte Unpack1/3 -> Model10/3
  Byte Unpack1/4 -> Model10/4
  UDP Receive1/1 -> Byte Unpack1/1

== system controller_dev_sg_HIL_noTP/Raptor State Machine 3 ==
  Enable : EnablePort
  Byte Unpack2 : etargetslib/Byte Unpack  dimensions={[1],[1],[1],[1]}  datatypes={'uint8','uint8','uint8','uint8'}  byteAlign=1
  Model11 : ModelReference  ModelNameDialog=RaptorStateMachine.slx  SimulationMode=Normal  ModelReferenceVersion=1.25
  Terminator2 : Terminator
  UDP Receive2 : xpcrtudplib/UDP Receive  ipAddressVal=10.0.0.20  localPort=ModCtrl_RaptorCommandVeh3_RcvPort  rcvWidth=4  rcvFmAny=on  fmAddress=10.0.0.1  rcvMulticast=off  multicastAddress={}  maxUDPQueue=8  sampleTime=-1
      settings: SourceProductName=Simulink Real-Time
  UDP Send3 : xpcrtudplib/UDP Send  ipAddressVal=10.0.0.20  localPort=40602  toAddress=10.0.0.13  toPort=ModCtrl_RaptorState_SendPort  sampleTime=-1
      settings: SourceProductName=Simulink Real-Time  SourceProductBaseCode=XP
  Width2 : Width
  wires:
  Byte Unpack2/4 -> Model11/4
  Model11/1 -> Width2/1, UDP Send3/1
  UDP Receive2/2 -> Terminator2/1
  Width2/1 -> UDP Send3/2
  Byte Unpack2/1 -> Model11/1
  Byte Unpack2/3 -> Model11/3
  UDP Receive2/1 -> Byte Unpack2/1
  Byte Unpack2/2 -> Model11/2

== system controller_dev_sg_HIL_noTP/Raptor State Machine 4 ==
  Enable : EnablePort
  Byte Unpack3 : etargetslib/Byte Unpack  dimensions={[1],[1],[1],[1]}  datatypes={'uint8','uint8','uint8','uint8'}  byteAlign=1
  Model12 : ModelReference  ModelNameDialog=RaptorStateMachine.slx  SimulationMode=Normal  ModelReferenceVersion=1.25
  Terminator6 : Terminator
  UDP Receive3 : xpcrtudplib/UDP Receive  ipAddressVal=10.0.0.20  localPort=ModCtrl_RaptorCommandVeh4_RcvPort  rcvWidth=4  rcvFmAny=on  fmAddress=10.0.0.1  rcvMulticast=off  multicastAddress={}  maxUDPQueue=8  sampleTime=-1
      settings: SourceProductName=Simulink Real-Time
  UDP Send4 : xpcrtudplib/UDP Send  ipAddressVal=10.0.0.20  localPort=40603  toAddress=10.0.0.14  toPort=ModCtrl_RaptorState_SendPort  sampleTime=-1
      settings: SourceProductName=Simulink Real-Time  SourceProductBaseCode=XP
  Width3 : Width
  wires:
  Byte Unpack3/2 -> Model12/2
  Byte Unpack3/4 -> Model12/4
  UDP Receive3/2 -> Terminator6/1
  UDP Receive3/1 -> Byte Unpack3/1
  Width3/1 -> UDP Send4/2
  Byte Unpack3/3 -> Model12/3
  Byte Unpack3/1 -> Model12/1
  Model12/1 -> Width3/1, UDP Send4/1

== system controller_dev_sg_HIL_noTP/Raptor State Machine 5 ==
  Enable : EnablePort
  Byte Unpack4 : etargetslib/Byte Unpack  dimensions={[1],[1],[1],[1]}  datatypes={'uint8','uint8','uint8','uint8'}  byteAlign=1
  Model13 : ModelReference  ModelNameDialog=RaptorStateMachine.slx  SimulationMode=Normal  ModelReferenceVersion=1.25
  Terminator7 : Terminator
  UDP Receive4 : xpcrtudplib/UDP Receive  ipAddressVal=10.0.0.20  localPort=ModCtrl_RaptorCommandVeh5_RcvPort  rcvWidth=4  rcvFmAny=on  fmAddress=10.0.0.1  rcvMulticast=off  multicastAddress={}  maxUDPQueue=8  sampleTime=-1
      settings: SourceProductName=Simulink Real-Time
  UDP Send5 : xpcrtudplib/UDP Send  ipAddressVal=10.0.0.20  localPort=40604  toAddress=10.0.0.15  toPort=ModCtrl_RaptorState_SendPort  sampleTime=-1
      settings: SourceProductName=Simulink Real-Time  SourceProductBaseCode=XP
  Width4 : Width
  wires:
  Width4/1 -> UDP Send5/2
  UDP Receive4/1 -> Byte Unpack4/1
  Model13/1 -> Width4/1, UDP Send5/1
  Byte Unpack4/2 -> Model13/2
  Byte Unpack4/3 -> Model13/3
  Byte Unpack4/1 -> Model13/1
  Byte Unpack4/4 -> Model13/4
  UDP Receive4/2 -> Terminator7/1

== system controller_dev_sg_HIL_noTP/Raptor State Machine 6 ==
  Enable : EnablePort
  Byte Unpack5 : etargetslib/Byte Unpack  dimensions={[1],[1],[1],[1]}  datatypes={'uint8','uint8','uint8','uint8'}  byteAlign=1
  Model14 : ModelReference  ModelNameDialog=RaptorStateMachine.slx  SimulationMode=Normal  ModelReferenceVersion=1.25
  Terminator8 : Terminator
  UDP Receive5 : xpcrtudplib/UDP Receive  ipAddressVal=10.0.0.20  localPort=ModCtrl_RaptorCommandVeh6_RcvPort  rcvWidth=4  rcvFmAny=on  fmAddress=10.0.0.1  rcvMulticast=off  multicastAddress={}  maxUDPQueue=8  sampleTime=-1
      settings: SourceProductName=Simulink Real-Time
  UDP Send6 : xpcrtudplib/UDP Send  ipAddressVal=10.0.0.20  localPort=40605  toAddress=10.0.0.16  toPort=ModCtrl_RaptorState_SendPort  sampleTime=-1
      settings: SourceProductName=Simulink Real-Time  SourceProductBaseCode=XP
  Width5 : Width
  wires:
  UDP Receive5/1 -> Byte Unpack5/1
  Width5/1 -> UDP Send6/2
  Byte Unpack5/2 -> Model14/2
  Model14/1 -> Width5/1, UDP Send6/1
  Byte Unpack5/1 -> Model14/1
  Byte Unpack5/3 -> Model14/3
  Byte Unpack5/4 -> Model14/4
  UDP Receive5/2 -> Terminator8/1

== system controller_dev_sg_HIL_noTP/Raptor State Machine 7 ==
  Enable : EnablePort
  Byte Unpack6 : etargetslib/Byte Unpack  dimensions={[1],[1],[1],[1]}  datatypes={'uint8','uint8','uint8','uint8'}  byteAlign=1
  Model15 : ModelReference  ModelNameDialog=RaptorStateMachine.slx  SimulationMode=Normal  ModelReferenceVersion=1.25
  Terminator9 : Terminator
  UDP Receive6 : xpcrtudplib/UDP Receive  ipAddressVal=10.0.0.20  localPort=ModCtrl_RaptorCommandVeh7_RcvPort  rcvWidth=4  rcvFmAny=on  fmAddress=10.0.0.1  rcvMulticast=off  multicastAddress={}  maxUDPQueue=8  sampleTime=-1
      settings: SourceProductName=Simulink Real-Time
  UDP Send7 : xpcrtudplib/UDP Send  ipAddressVal=10.0.0.20  localPort=40606  toAddress=10.0.0.17  toPort=ModCtrl_RaptorState_SendPort  sampleTime=-1
      settings: SourceProductName=Simulink Real-Time  SourceProductBaseCode=XP
  Width6 : Width
  wires:
  UDP Receive6/2 -> Terminator9/1
  Byte Unpack6/4 -> Model15/4
  Byte Unpack6/1 -> Model15/1
  Byte Unpack6/2 -> Model15/2
  UDP Receive6/1 -> Byte Unpack6/1
  Model15/1 -> Width6/1, UDP Send7/1
  Byte Unpack6/3 -> Model15/3
  Width6/1 -> UDP Send7/2

== system controller_dev_sg_HIL_noTP/Raptor State Machine 8 ==
  Enable : EnablePort
  Byte Unpack7 : etargetslib/Byte Unpack  dimensions={[1],[1],[1],[1]}  datatypes={'uint8','uint8','uint8','uint8'}  byteAlign=1
  Model16 : ModelReference  ModelNameDialog=RaptorStateMachine.slx  SimulationMode=Normal  ModelReferenceVersion=1.25
  Terminator10 : Terminator
  UDP Receive7 : xpcrtudplib/UDP Receive  ipAddressVal=10.0.0.20  localPort=ModCtrl_RaptorCommandVeh8_RcvPort  rcvWidth=4  rcvFmAny=on  fmAddress=10.0.0.1  rcvMulticast=off  multicastAddress={}  maxUDPQueue=8  sampleTime=-1
      settings: SourceProductName=Simulink Real-Time
  UDP Send8 : xpcrtudplib/UDP Send  ipAddressVal=10.0.0.20  localPort=40607  toAddress=10.0.0.18  toPort=ModCtrl_RaptorState_SendPort  sampleTime=-1
      settings: SourceProductName=Simulink Real-Time  SourceProductBaseCode=XP
  Width7 : Width
  wires:
  UDP Receive7/2 -> Terminator10/1
  Model16/1 -> Width7/1, UDP Send8/1
  UDP Receive7/1 -> Byte Unpack7/1
  Byte Unpack7/1 -> Model16/1
  Byte Unpack7/4 -> Model16/4
  Byte Unpack7/3 -> Model16/3
  Byte Unpack7/2 -> Model16/2
  Width7/1 -> UDP Send8/2

== system controller_dev_sg_HIL_noTP/Rx_VehicleControlCAN ==
  CAN Read : speedgoatlib_IO612/CAN Read  id=1  sampleTime=-1  portSelection=1  messageType=CAN  protl=IO612  ptIdx=0  isFDMod=0
      settings: SourceProductName=Simulink Real-Time: Speedgoat I/O Driver Library
  CAN Unpack : canmsglib/CAN Unpack  MsgList=(none)  MsgName=CAN Msg  MsgIDType=Standard (11-bit identifier)  MsgIdentifier=24  MsgLength=8  SignalInfo=SteeringAngleAtWheel_rad$0$24$1$1$1$0$0.000001$0$-Inf$Inf$#TractionforceSummedAtWheels_N$24$24$1$1$1$0$0.01$0$-Inf$Inf$#  NSignals=2  IDPort=off  TimestampPort=off  ErrorPort=off  RemotePort=off  LengthPort=off  StatusPort=off  StartBits=str2num('[int32(0);int32(24)]')  SignalSizes=str2num('[int32(24);int32(24)]')  ByteOrders=str2num('[int32(1);int32(1)]')  DataTypes=str2num('[int32(1);int32(1)]')  MultiplexTypes=str2num('[int32(1);int32(1)]')  MultiplexValues=str2num('[double(0);double(0)]')  Factors=str2num('[double(0.000001);double(0.01)]')  Offsets=str2num('[double(0);double(0)]')  Minimums=str2num('[double(-Inf);double(-Inf)]')  Maximums=str2num('[double(Inf);double(Inf)]')  ApplyMinMax=off
      settings: SourceProductName=Simulink Real-Time
  While Iterator : WhileIterator  MaxIters=501  WhileBlockType=do-while
  SteeringAngleAtWheel_rad : Outport
  TractionForceSummedAtWheels_N : Outport  Port=2
  wires:
  CAN Unpack/2 -> TractionForceSummedAtWheels_N/1
  CAN Unpack/1 -> SteeringAngleAtWheel_rad/1
  CAN Read/2 -> CAN Unpack/1
  CAN Read/1 -> While Iterator/1
